simulink model "lab_03_convolution"  (R2024b)
settings: Solver=VariableStepAuto  StartTime=0.0  StopTime=10.0  RelTol=1e-3
settings Model: LastModifiedBy=LENOVO

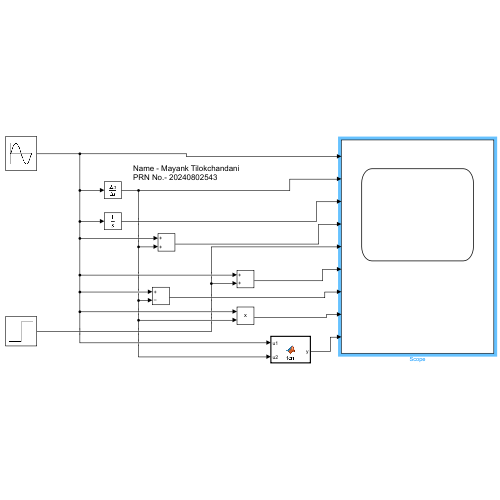
[thumbnail: Simulink's stored preview of the top-level diagram]
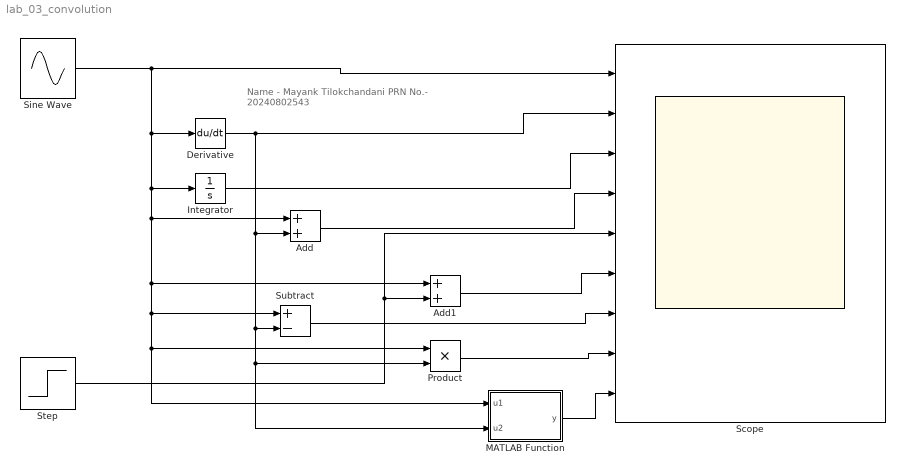
== system lab_03_convolution ==
  note: Name - Mayank Tilokchandani
      | PRN No.- 20240802543
  Add : Sum
  Add1 : Sum
  Derivative : Derivative
  Integrator : Integrator
  MATLAB Function : MATLAB Function  TreatAsAtomicUnit=on
  Product : Product
  Scope : Scope  NumInputPorts=9
  Sine Wave : Sin  SampleTime=0
  Step : Step  SampleTime=0
  Subtract : Sum  Inputs=+-
  wires:
  Sine Wave/1 -> Product/1, MATLAB Function/1(u1), Subtract/1, Add1/1, Add/1, Integrator/1, Derivative/1, Scope/1
  Derivative/1 -> Product/2, MATLAB Function/2(u2), Subtract/2, Add/2, Scope/2
  Integrator/1 -> Scope/3
  Add/1 -> Scope/4
  Step/1 -> Scope/5, Add1/2
  Add1/1 -> Scope/6
  Subtract/1 -> Scope/7
  Product/1 -> Scope/8
  MATLAB Function/1(y) -> Scope/9

== matlab function lab_03_convolution/MATLAB Function ==
  data: u1 input; y output; u2 input
function y = fcn(u1,u2)

y = conv(u1,u2);
